simulink model "Signalflussplan"  (R2016b)
settings: Solver=VariableStepAuto  StartTime=0.0  StopTime=10.0  RelTol=1e-3
undefined symbols (not defined in the file): c, m, n
libraries: hdlsllib x6
settings Model: Creator=Anton  LastModifiedBy=Anton

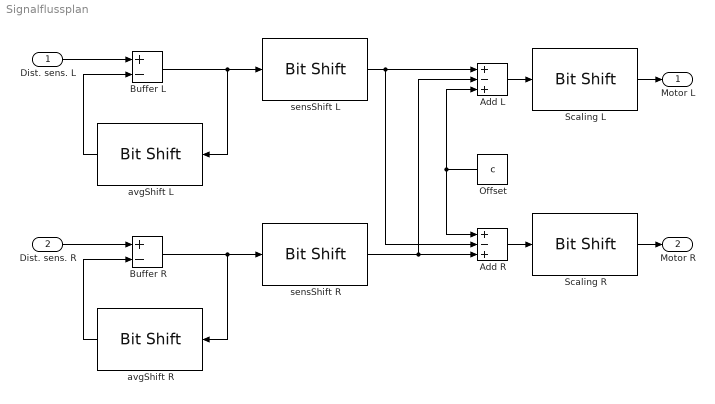
== system Signalflussplan ==
  Dist. sens. L : Inport
  Dist. sens. R : Inport  Port=2
  Add L : Sum  Inputs=+-+
  Add R : Sum  Inputs=+-+
  Buffer L : Sum  Inputs=+-
  "Buffer R " : Sum  Inputs=+-
  Offset : Constant  Value=c
  Scaling L : hdlsllib/HDL Operations/Bit Shift  mode=Shift Right Logical  N=1
  Scaling R : hdlsllib/HDL Operations/Bit Shift  mode=Shift Right Logical  N=1
  "avgShift L " : hdlsllib/HDL Operations/Bit Shift  mode=Shift Right Logical  N=n
  avgShift R : hdlsllib/HDL Operations/Bit Shift  mode=Shift Right Logical  N=n
  sensShift L : hdlsllib/HDL Operations/Bit Shift  mode=Shift Right Logical  N=n + m
  sensShift R : hdlsllib/HDL Operations/Bit Shift  mode=Shift Right Logical  N=n + m
  Motor L : Outport
  Motor R : Outport  Port=2
  wires:
  Dist. sens. L/1 -> Buffer L/1
  Buffer L/1 -> sensShift L/1, "avgShift L "/1
  "avgShift L "/1 -> Buffer L/2
  Dist. sens. R/1 -> "Buffer R "/1
  "Buffer R "/1 -> sensShift R/1, avgShift R/1
  avgShift R/1 -> "Buffer R "/2
  sensShift L/1 -> Add R/2, Add L/1
  Offset/1 -> Add R/1, Add L/3
  sensShift R/1 -> Add L/2, Add R/3
  Add L/1 -> Scaling L/1
  Scaling L/1 -> Motor L/1
  Add R/1 -> Scaling R/1
  Scaling R/1 -> Motor R/1
